simulink model "msd03_SimulinkModeling"  (R2025b)
settings: Solver=VariableStepAuto  StartTime=0.0  StopTime=10.0  MaxStep=0.01  RelTol=1e-3
InitFcn:
  | m=3.6;
  | k=400;
  | b = 10;
settings Model: Creator=ayeo  LastModifiedBy=ayeo

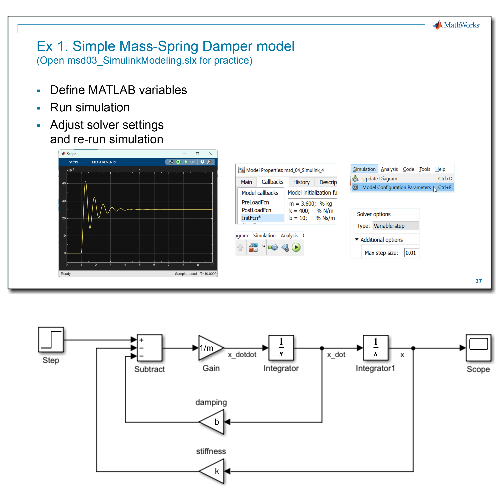
[thumbnail: Simulink's stored preview of the top-level diagram]
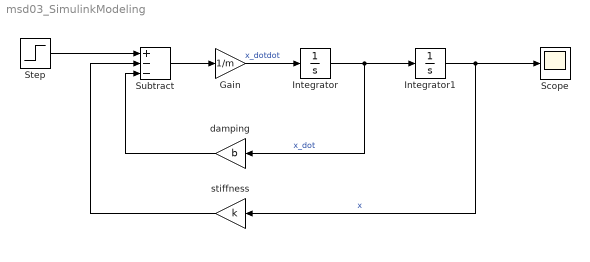
== system msd03_SimulinkModeling ==
  Gain : Gain  Gain=1/m
  Integrator : Integrator
  Integrator1 : Integrator
  Scope : Scope
      settings: ActiveDisplayYMinimum=-0.00051831926479820576  ActiveDisplayYMaximum=0.0046648733831838526
  Step : Step  SampleTime=0
  Subtract : Sum  Inputs=+--
  damping : Gain  Gain=b
  stiffness : Gain  Gain=k
  wires:
  Integrator/1 -> damping/1, Integrator1/1  "x_dot"
  Gain/1 -> Integrator/1  "x_dotdot"
  Integrator1/1 -> Scope/1, stiffness/1  "x"
  Subtract/1 -> Gain/1
  Step/1 -> Subtract/1
  damping/1 -> Subtract/3
  stiffness/1 -> Subtract/2
